simulink model "PlanemodelRelay"  (R2016b)
settings: Solver=ode15s  StartTime=0.0  StopTime=10  MaxStep=0.1  RelTol=1e-3  AbsTol=1e-3
values from neighbouring files (symbols this model uses):
  Kf = 1.27*[1 1]    [design4.m]
  T_f = 0.28    [design4.m]
undefined symbols (not defined in the file or in its folder): A, B, C, D
undefined symbols (not defined in the file): Ctheta, L
settings Model: ExtModeTrigMode=oneshot  ExtModeArmWhenConnect=off  Creator=sven  LastModifiedBy=peyam
settings DataIOCC: SaveFormat=Array  SignalLoggingSaveFormat=ModelDataLogs  SaveOutput=off  SaveTime=off
settings OptimizationCC: BlockReduction=off  BooleanDataType=off
settings DebuggingCC: SaveWithParameterizedLinksMsg=none  UnderspecifiedInitializationDetection=Classic  MergeDetectMultiDrivingBlocksExec=none  SignalResolutionControl=TryResolveAllWithWarning  MultiTaskDSMMsg=warning  MultiTaskCondExecSysMsg=none
settings HardwareCC: TargetUnknown=on
settings ModelReferenceCC: PropagateSignalLabelsOutOfModel=off
settings RTWCC: TemplateMakefile=grt_unix.tmf
settings GRTTargetCC: TargetLangStandard=C89/C90 (ANSI)  CombineOutputUpdateFcns=off  GRTInterface=on

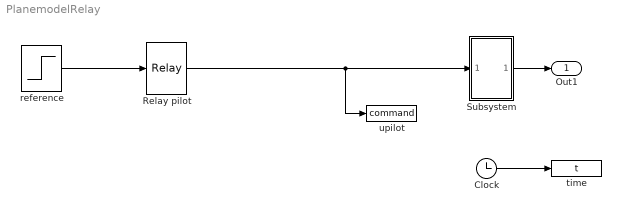
== system PlanemodelRelay ==
  Clock : Clock
  Relay pilot : Relay  OffSwitchValue=-eps  OnOutputValue=0.2  OffOutputValue=-0.2
  Subsystem : Subsystem
  reference : Step  Time=0  SampleTime=0
  time : ToWorkspace  VariableName=t
      settings: MaxDataPoints=10000
  upilot : ToWorkspace  VariableName=command
      settings: MaxDataPoints=10000
  Out1 : Outport
  wires:
  Clock/1 -> time/1
  reference/1 -> Relay pilot/1
  Relay pilot/1 -> upilot/1, Subsystem/1(In1)
  Subsystem/1(Out1) -> Out1/1

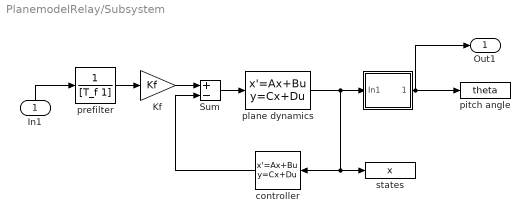
== system PlanemodelRelay/Subsystem ==
  In1 : Inport
  " " : Subsystem  mask(Matrix Gain){K=Ctheta}
      mask prompts: K "Gain matrix:"
      mask help: Matrix Gain.
      mask Help: Multiplies input vector by entered matrix to produce output vector (y=Au).
      mask Display: disp('Ctheta')
  Kf : Gain  Gain=Kf  SaturateOnIntegerOverflow=on  OutDataTypeStr=Inherit: Same as input  ParamDataTypeStr=Inherit: Same as input
  Sum : Sum  Inputs=+-  SaturateOnIntegerOverflow=on  InputSameDT=on  OutDataTypeStr=Inherit: Same as first input
  controller : StateSpace  A=[]  B=[]  C=[]  D=K  X0=0  mask(Matrix gain){K=L}
      mask prompts: K "Gain matrix:"
      mask help: Matrix Gain:
      mask Help: Multiplies input vector by entered matrix to produce output vector.
      mask Display: disp('L')
  pitch angle : ToWorkspace  VariableName=theta
      settings: MaxDataPoints=10000
  plane dynamics : StateSpace  A=A  B=B  C=C  D=D  X0=0
  prefilter : TransferFcn  Denominator=[T_f 1]
  states : ToWorkspace  VariableName=x
      settings: MaxDataPoints=10000
  Out1 : Outport
  wires:
  Sum/1 -> plane dynamics/1
  prefilter/1 -> Kf/1
  plane dynamics/1 -> " "/1(In1), controller/1, states/1
  controller/1 -> Sum/2
  " "/1(Out1) -> Out1/1, pitch angle/1
  Kf/1 -> Sum/1
  In1/1 -> prefilter/1

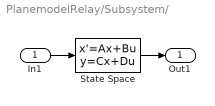
== system PlanemodelRelay/Subsystem/  ==
  In1 : Inport
  State Space : StateSpace  A=[]  B=[]  C=[]  D=K  X0=0
  Out1 : Outport
  wires:
  In1/1 -> State Space/1
  State Space/1 -> Out1/1
